simulink model "Assignment_TestGen12"  (R2017b)
settings: Solver=FixedStepDiscrete  StartTime=0.0  StopTime=10.0  RelTol=1e-3
undefined symbols (not defined in the file): Block_TestLib, enable
settings Model: Creator=hbourbou  LastModifiedBy=hbourbou
settings DebuggingCC: ParameterOverflowMsg=none

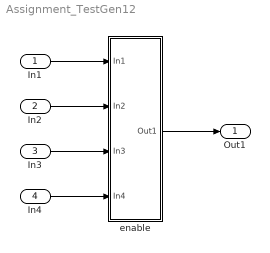
== system Assignment_TestGen12 ==
  In1 : Inport
  In2 : Inport  Port=2
  In3 : Inport  Port=3
  In4 : Inport  Port=4
  enable : Subsystem  AncestorBlock=Block_TestLib/enable
  Out1 : Outport
  wires:
  In1/1 -> enable/1(In1)
  In2/1 -> enable/2(In2)
  In3/1 -> enable/3(In3)
  In4/1 -> enable/4(In4)
  enable/1(Out1) -> Out1/1

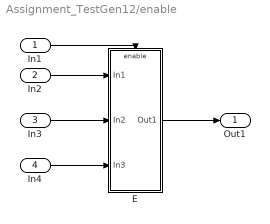
== system Assignment_TestGen12/enable ==
  In1 : Inport  OutDataTypeStr=boolean
  In2 : Inport  Port=2
  In3 : Inport  Port=3
  In4 : Inport  Port=4
  E : Subsystem  TreatAsAtomicUnit=on
  Out1 : Outport
  wires:
  In1/1 -> E/Enable
  In2/1 -> E/1(In1)
  In3/1 -> E/2(In2)
  In4/1 -> E/3(In3)
  E/1(Out1) -> Out1/1

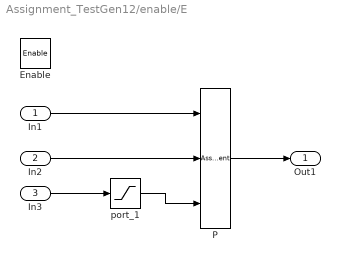
== system Assignment_TestGen12/enable/E ==
  In1 : Inport  OutDataTypeStr=double  PortDimensions=[3 3 3]
  In2 : Inport  Port=2  OutDataTypeStr=double  PortDimensions=[2 2 2]
  In3 : Inport  Port=3  OutMin=1  OutMax=2
  Enable : EnablePort
  P : Assignment  NumberOfDimensions=3  DiagnosticForDimensions=Warning  IndexOptions=Index vector (dialog),Index vector (port),Starting index (dialog)  Indices=[1,2],[],1  OutputSizes=,,
  port_1 : Saturate  UpperLimit=2  LowerLimit=1
  Out1 : Outport
  wires:
  In1/1 -> P/1
  In2/1 -> P/2
  port_1/1 -> P/3
  In3/1 -> port_1/1
  P/1 -> Out1/1
